simulink model "autopilot_waypoint_mission"  (R2025b)
settings: Solver=FixedStepAuto  StartTime=0.0  StopTime=400  FixedStep=0.01  RelTol=1e-3
InitFcn:
  | %% environmental parameter
  | 
  | g = 9.81;                       %[m/ss]
  | 
  | %% Vehicle parameter
  | 
  | mass = 1.5;                     %[kg]
  | Arm_Length = 0.225;             %[m]
  | 
  | %% Motor parameter
  | 
  | rad2rpm = 60 / (2 * pi);
  | 
  | rpm2rad = 1 / rad2rpm;
  | 
  | Friction_Coef = 0.0001;         %[N m /s]
  | 
  | Inertia = 2.8e-05;              %[kg m^2]
  | 
  | Resistance = 0.1170;            %[ohm]
  | 
  | K_Torque = 1 / (rpm2rad * 960); %[N m/A]
  | 
  | K_Emf = K_Torque;               %[V s/rad]
  | 
  | tau = (Inertia * Resistance) / (Resistance * Friction_Coef + K_Torque * K_Emf);
  | 
  | k_s = K_Torque / (Resistance * Friction_Coef + K_Torque * K_Emf);
  | 
  | Thrust_Coef = 1.1768e-05;
  | 
  | Drag_Coef = 1.8542e-07;
  | 
  | Hovering_Motor_Speed = sqrt(mass * g / (4 * Thrust_Coef));
  | 
  | k_p = 1/k_s;
  | 
  | K1_ALT = 2.1;
  | K2_ALT = 0.7142;
  | 
  | K1_POS = 1.26;
  | K2_POS = 0.4286;
libraries: simulink_extras x8, uavutilslib x1
settings Model: Creator=user  LastModifiedBy=user

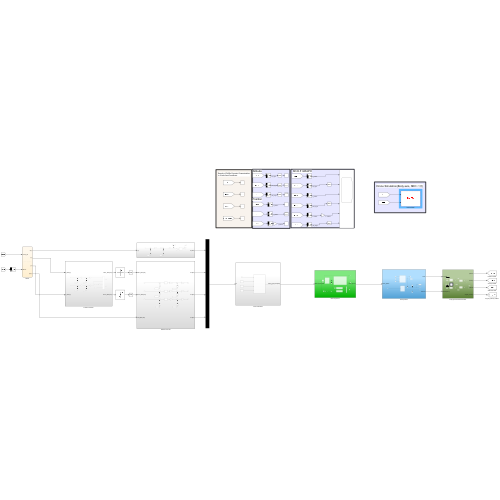
[thumbnail: Simulink's stored preview of the top-level diagram]
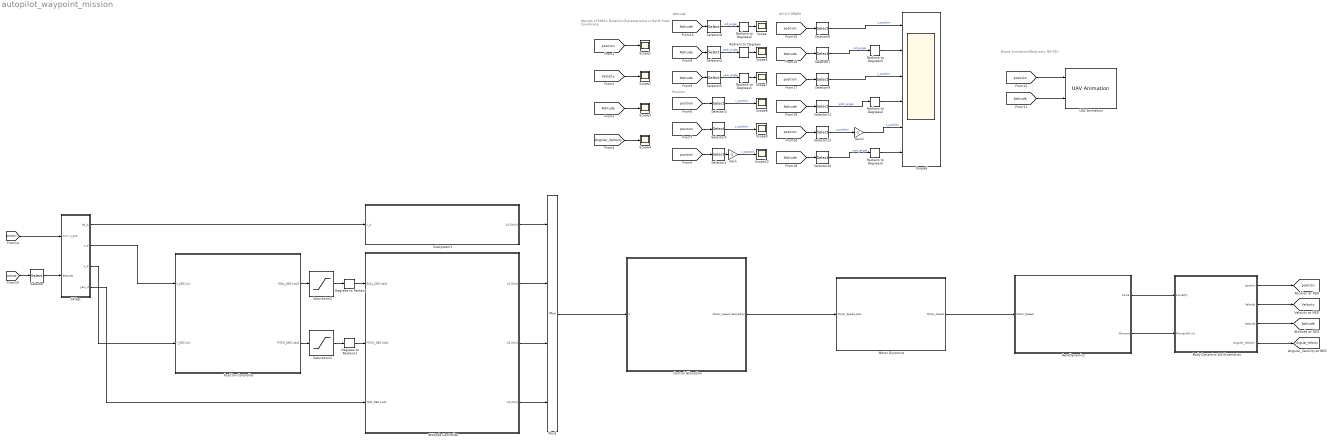
== system autopilot_waypoint_mission ==
  note: Attitude
  note: Results of F450's Dynamic Characteristics
      | in Earth fixed Coordinate
  note: Position
  note: 6D.O.F GRAPH
  note: Drone Simulation(Body axis, NED 기준)
  AeroDynamics : Subsystem
  Attitude Controller : Subsystem
  Body Dynamics && Kinematics : Subsystem
  Control Allocation : Subsystem
  Degrees to Radians : simulink_extras/Transformations/Degrees to Radians
  Degrees to Radians1 : simulink_extras/Transformations/Degrees to Radians
  Gain : Gain  Gain=-1
  Gain1 : Gain  Gain=-1
  Motor Dynamics : Subsystem
  Mux1 : Mux
  Position Controller : Subsystem
  Radians to Degrees{,1..5} (6 alike) : simulink_extras/Transformations/Radians to Degrees
  SP Set : Stateflow chart  TreatAsAtomicUnit=on
      settings: PortSchema="{\"entries\":[{\"content\":{\"sides\":[{\"content\":{},\"type\":\"ConnectorPlacement.EquallySpacedRectSide\",\"uuid\":\"3e53484f-0db2-495f-837b-267abd105f28\"},{\"content\":{\"side\":\"RIGHT\"},\"type\":\"ConnectorPlacement.EquallySpacedRectSide\",\"uuid\":\"c216aad6-ad66-4255-85c0-6c38f2606c75\"},{\"content\":{\"connectorIds\":[\"In2\",\"In1\"],\"side\":\"TOP\"},\"type\":\"ConnectorPlacement.EquallySpacedRectSide\",\"uuid\":\"2b1aea76-ce92-43d3-9c38-2c398ee5c197\"},{\"content\":{\"connectorIds\":[\"Out4\",\"Out2\",\"Out1\",\"Out3\"],\"side\":\"BOTTOM\"},\"type\":\"ConnectorPlacement.EquallySpacedRectSide\",\"uuid\":\"b9774cfe-4d99-465a-9e54-dae465952399\"}]},\"type\":\"ConnectorPlacement.EquallySpacedConnector\",\"uuid\":\"ddf8ca19-aa2c-423c-a9ec-aafb509ad8aa\"}],\"packageUris\":[\"http://schema.mathworks.com/mf0/Connector/R2020b\"],\"version\":\"1.0\"}"
  Saturation1 : Saturate  UpperLimit=30  LowerLimit=-30
  Saturation2 : Saturate  UpperLimit=30  LowerLimit=-30
  Scope{,1..5,7..10} (10 alike) : Scope
      Scope1 settings: Title=Position  ActiveDisplayYMinimum=-2599.70657  ActiveDisplayYMaximum=308.02028  YLabel=[m]  DataLoggingVariableName=ScopeData2
      Scope10 settings: DataLoggingVariableName=ScopeData6
      Scope2 settings: Title=Velocity  ActiveDisplayYMinimum=-56.12917  ActiveDisplayYMaximum=85.41613  YLabel=[m/s]  DataLoggingVariableName=ScopeData3
      Scope3 settings: Title=Attitude  ActiveDisplayYMinimum=-0.68224  ActiveDisplayYMaximum=0.69065  YLabel=[rad]
      Scope4 settings: Title=Angular_Velocity  ActiveDisplayYMinimum=-2.51743  ActiveDisplayYMaximum=2.43948  YLabel=[rad/s]  DataLoggingVariableName=ScopeData2
      Scope5 settings: DataLoggingVariableName=ScopeData2
      Scope7 settings: ActiveDisplayYMinimum=-114.67339  ActiveDisplayYMaximum=12.74149  DataLoggingVariableName=ScopeData3
      Scope8 settings: DataLoggingVariableName=ScopeData4
      Scope9 settings: DataLoggingVariableName=ScopeData5
  Scope6 : Scope  NumInputPorts=6
      settings: ActiveDisplayYMinimum=-3713.64731  ActiveDisplayYMaximum=1009.89473
  Selector : Selector  InputPortWidth=3  IndexOptions=Index vector (dialog)  Indices=3  OutputSizes=1
  Selector{1,5,9..10} (4 alike) : Selector  InputPortWidth=3  IndexOptions=Index vector (dialog)  Indices=[3]  OutputSizes=1
  Selector{2,6,8,11} (4 alike) : Selector  InputPortWidth=3  IndexOptions=Index vector (dialog)  Indices=1  OutputSizes=1
  Selector12 : Selector  InputPortWidth=3  IndexOptions=Index vector (dialog)  Indices=3  OutputSizes=1
  Selector3 : Selector  InputPortWidth=3  IndexOptions=Index vector (dialog)  Indices=2  OutputSizes=1
  Selector4 : Selector  InputPortWidth=3  IndexOptions=Index vector (dialog)  Indices=2  OutputSizes=1
  Selector7 : Selector  InputPortWidth=3  IndexOptions=Index vector (dialog)  Indices=2  OutputSizes=1
  Subsystem1 : Subsystem
  UAV Animation : uavutilslib/UAV Animation  NumUAV=1  DynamicUAVConfig=off  UAVType=Multirotor  UAVSize=1  UAVColor=[1 0 0]  UAVTrajectoryAlpha=1  InertialZDirection=Down  RotationFormat=Euler ZYX  DrawMarkers=off  SampleTime=0.1
  tag scope: Angular_Velocity=global, Attitude=global, Velocity=global, position=global
  wires:
  Motor Dynamics/1(Motor_Speed) -> AeroDynamics/1(Motor_Speed)
  Body Dynamics && Kinematics/3(attitude) -> [Attitude]
  Body Dynamics && Kinematics/1(position) -> [position]
  [Velocity] -> Scope2/1
  [position] -> Scope1/1
  AeroDynamics/1(Force) -> Body Dynamics && Kinematics/1(Force[N])
  AeroDynamics/2(Moment) -> Body Dynamics && Kinematics/2(Moment[N m])
  Body Dynamics && Kinematics/2(Velocity) -> [Velocity]
  Body Dynamics && Kinematics/4(Angular_Velocity) -> [Angular_Velocity]
  [Attitude] -> Scope3/1
  [Angular_Velocity] -> Scope4/1
  Control Allocation/1(Motor_speed_des[rad/s]) -> Motor Dynamics/1(Motor_Speed_Des)
  Mux1/1 -> Control Allocation/1(U)
  [Attitude] -> Selector8/1
  Attitude Controller/1(U2 [Nm]) -> Mux1/2
  Attitude Controller/2(U3 [Nm]) -> Mux1/3
  Attitude Controller/3(U4 [Nm]) -> Mux1/4
  Subsystem1/1(U1 [N/m]) -> Mux1/1
  Selector1/1 -> Gain/1
  [position] -> Selector1/1
  Position Controller/1(ROLL_DES [rad]) -> Saturation2/1
  Position Controller/2(PITCH_DES [rad]) -> Saturation1/1
  [position] -> Selector2/1
  [position] -> Selector3/1
  [Attitude] -> Selector4/1
  [Attitude] -> Selector5/1
  Saturation1/1 -> Degrees to Radians1/1
  Degrees to Radians1/1 -> Attitude Controller/2(PITCH_DES [rad])
  Saturation2/1 -> Degrees to Radians/1
  Degrees to Radians/1 -> Attitude Controller/1(ROLL_DES [rad])
  SP Set/3(alt_d) -> Subsystem1/1(x_d)
  SP Set/1(x_d) -> Position Controller/1(X_DES [m])
  SP Set/2(y_d) -> Position Controller/2(Y_DES [m])
  SP Set/4(yaw_d) -> Attitude Controller/3(YAW_DES [rad])
  [position] -> SP Set/1(current_pos)
  [Attitude] -> Selector/1
  Selector/1 -> SP Set/2(attitude)
  [position] -> UAV Animation/1
  [Attitude] -> UAV Animation/2
  Selector8/1 -> Radians to Degrees2/1  "roll_angle"
  Selector4/1 -> Radians to Degrees/1  "pitch_angle"
  Selector5/1 -> Radians to Degrees1/1  "yaw_angle"
  Selector2/1 -> Scope8/1  "x_position"
  Selector3/1 -> Scope9/1  "y_position"
  Gain/1 -> Scope10/1  "z_position"
  Selector6/1 -> Scope6/1  "x_position"
  [position] -> Selector6/1
  Selector9/1 -> Scope6/3  "y_position"
  Selector7/1 -> Radians to Degrees3/1  "roll_angle"
  [position] -> Selector9/1
  [Attitude] -> Selector7/1
  Selector12/1 -> Gain1/1  "z_position"
  Selector10/1 -> Radians to Degrees5/1  "yaw_angle"
  Selector11/1 -> Radians to Degrees4/1  "pitch_angle"
  [Attitude] -> Selector10/1
  [position] -> Selector12/1
  [Attitude] -> Selector11/1
  Gain1/1 -> Scope6/5  "z_position"
  Radians to Degrees/1 -> Scope5/1
  Radians to Degrees1/1 -> Scope7/1
  Radians to Degrees2/1 -> Scope/1
  Radians to Degrees3/1 -> Scope6/2
  Radians to Degrees4/1 -> Scope6/4
  Radians to Degrees5/1 -> Scope6/6

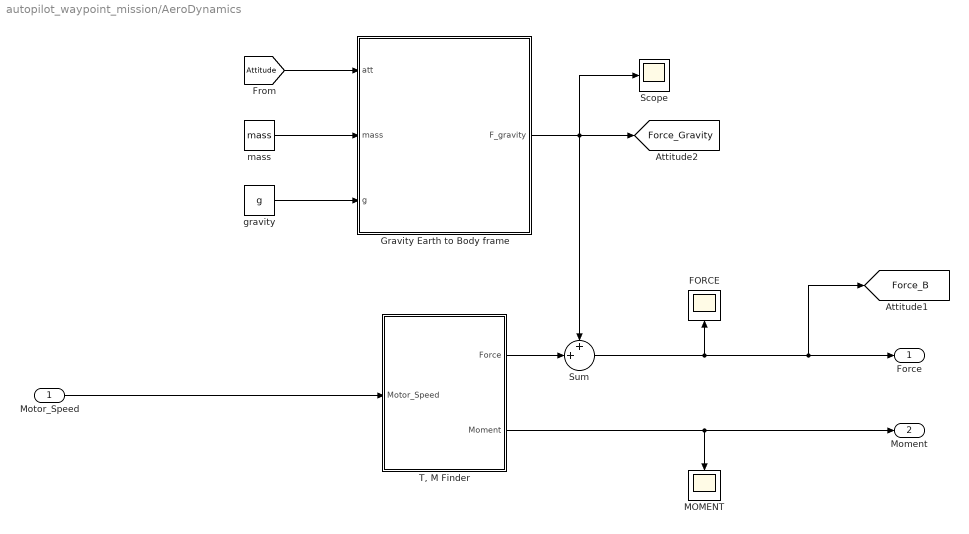
== system autopilot_waypoint_mission/AeroDynamics ==
  Motor_Speed : Inport
  FORCE : Scope
      settings: Title=Body Force Net  ActiveDisplayYMinimum=-2.48819  ActiveDisplayYMaximum=16.62647  YLabel=Force [N]  DataLoggingVariableName=ScopeData4
  Gravity Earth to Body frame : MATLAB Function  TreatAsAtomicUnit=on
  MOMENT : Scope
      settings: ActiveDisplayYMinimum=-0.01497  ActiveDisplayYMaximum=0.13326  DataLoggingVariableName=ScopeData5
  Scope : Scope
      settings: Title=Force_gravity in NED  ActiveDisplayYMinimum=-1.83938  ActiveDisplayYMaximum=16.55438  YLabel=Force [N]
  Sum : Sum  Inputs=++|
  "T, M Finder" : MATLAB Function  TreatAsAtomicUnit=on
  gravity : Constant  Value=g
  mass : Constant  Value=mass
  Force : Outport
  Moment : Outport  Port=2
  tag scope: Force_B=global, Force_Gravity=global
  wires:
  [Attitude] -> Gravity Earth to Body frame/1(att)
  Gravity Earth to Body frame/1(F_gravity) -> Scope/1, [Force_Gravity], Sum/1
  Motor_Speed/1 -> "T, M Finder"/1(Motor_Speed)
  mass/1 -> Gravity Earth to Body frame/2(mass)
  "T, M Finder"/1(Force) -> Sum/2
  gravity/1 -> Gravity Earth to Body frame/3(g)
  Sum/1 -> [Force_B], Force/1, FORCE/1
  "T, M Finder"/2(Moment) -> Moment/1, MOMENT/1

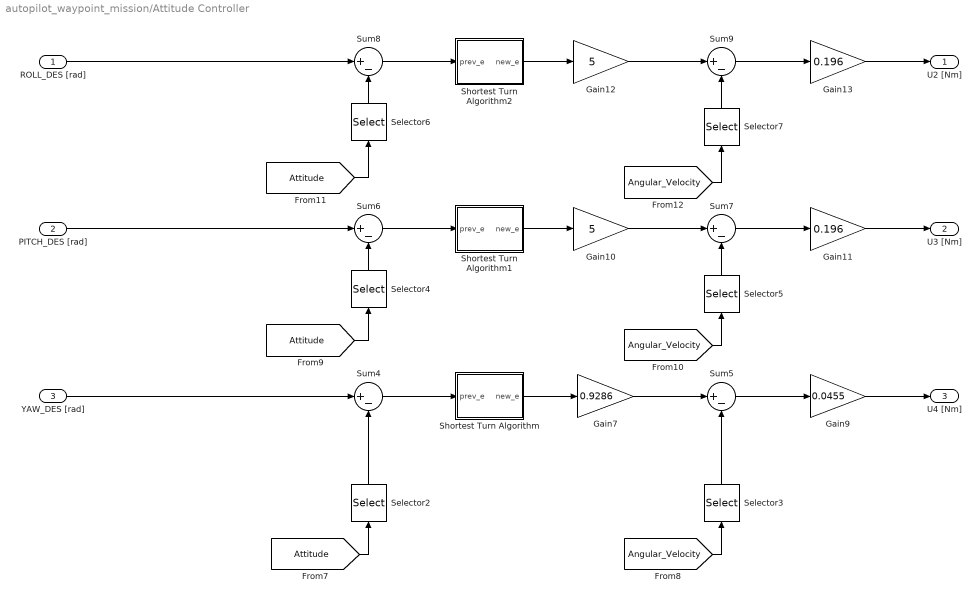
== system autopilot_waypoint_mission/Attitude Controller ==
  ROLL_DES [rad] : Inport
  PITCH_DES [rad] : Inport  Port=2
  YAW_DES [rad] : Inport  Port=3
  Gain10 : Gain  Gain=5
  Gain11 : Gain  Gain=0.196
  Gain12 : Gain  Gain=5
  Gain13 : Gain  Gain=0.196
  Gain7 : Gain  Gain=0.9286
  Gain9 : Gain  Gain=0.0455
  Selector2 : Selector  InputPortWidth=3  IndexOptions=Index vector (dialog)  Indices=[3]  OutputSizes=1
  Selector3 : Selector  InputPortWidth=3  IndexOptions=Index vector (dialog)  Indices=[3]  OutputSizes=1
  Selector4 : Selector  InputPortWidth=3  IndexOptions=Index vector (dialog)  Indices=[2]  OutputSizes=1
  Selector5 : Selector  InputPortWidth=3  IndexOptions=Index vector (dialog)  Indices=[2]  OutputSizes=1
  Selector6 : Selector  InputPortWidth=3  IndexOptions=Index vector (dialog)  Indices=[1]  OutputSizes=1
  Selector7 : Selector  InputPortWidth=3  IndexOptions=Index vector (dialog)  Indices=[1]  OutputSizes=1
  Shortest Turn Algorithm : MATLAB Function  TreatAsAtomicUnit=on
  Shortest Turn Algorithm1 : MATLAB Function  TreatAsAtomicUnit=on
  Shortest Turn Algorithm2 : MATLAB Function  TreatAsAtomicUnit=on
  Sum{4..9} (6 alike) : Sum  Inputs=|+-
  U2 [Nm] : Outport
  U3 [Nm] : Outport  Port=2
  U4 [Nm] : Outport  Port=3
  wires:
  Shortest Turn Algorithm/1(new_e) -> Gain7/1
  Gain9/1 -> U4 [Nm]/1
  [Attitude] -> Selector4/1
  Selector4/1 -> Sum6/2
  [Angular_Velocity] -> Selector3/1
  Gain7/1 -> Sum5/1
  Selector6/1 -> Sum8/2
  Sum9/1 -> Gain13/1
  Gain12/1 -> Sum9/1
  Gain10/1 -> Sum7/1
  Selector5/1 -> Sum7/2
  Sum4/1 -> Shortest Turn Algorithm/1(prev_e)
  [Angular_Velocity] -> Selector7/1
  Sum7/1 -> Gain11/1
  PITCH_DES [rad]/1 -> Sum6/1
  Selector2/1 -> Sum4/2
  [Angular_Velocity] -> Selector5/1
  Gain11/1 -> U3 [Nm]/1
  Selector3/1 -> Sum5/2
  [Attitude] -> Selector6/1
  ROLL_DES [rad]/1 -> Sum8/1
  [Attitude] -> Selector2/1
  Sum5/1 -> Gain9/1
  Selector7/1 -> Sum9/2
  YAW_DES [rad]/1 -> Sum4/1
  Gain13/1 -> U2 [Nm]/1
  Sum8/1 -> Shortest Turn Algorithm2/1(prev_e)
  Shortest Turn Algorithm2/1(new_e) -> Gain12/1
  Sum6/1 -> Shortest Turn Algorithm1/1(prev_e)
  Shortest Turn Algorithm1/1(new_e) -> Gain10/1

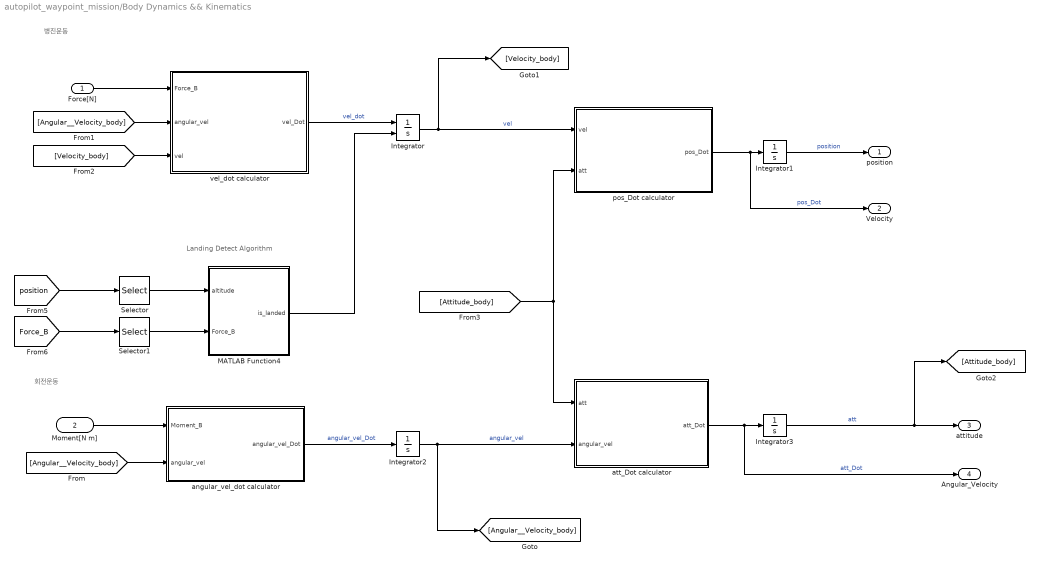
== system autopilot_waypoint_mission/Body Dynamics && Kinematics ==
  note: 병진운동
  note: 회전운동
  note: Landing Detect Algorithm
  Force[N] : Inport
  Moment[N m] : Inport  Port=2
  Integrator : Integrator  ExternalReset=level hold  InitialCondition=[0 0 0]'
  Integrator1 : Integrator  InitialCondition=[0 0 0]'  LimitOutput=on  UpperSaturationLimit=[inf inf 0]'  LowerSaturationLimit=[-inf -inf -inf]'  ZeroCross=off
  Integrator2 : Integrator  InitialCondition=[0 0 0]'
  Integrator3 : Integrator  InitialCondition=[0 0 0]'  WrapState=on
  MATLAB Function4 : MATLAB Function  TreatAsAtomicUnit=on
  Selector : Selector  InputPortWidth=3  IndexOptions=Index vector (dialog)  Indices=[3]  OutputSizes=1
  Selector1 : Selector  InputPortWidth=3  IndexOptions=Index vector (dialog)  Indices=[3]  OutputSizes=1
  angular_vel_dot calculator : MATLAB Function  TreatAsAtomicUnit=on
  att_Dot calculator : MATLAB Function  TreatAsAtomicUnit=on
  pos_Dot calculator : MATLAB Function  TreatAsAtomicUnit=on
  vel_dot calculator : MATLAB Function  TreatAsAtomicUnit=on
  position : Outport
  Velocity : Outport  Port=2
  attitude : Outport  Port=3
  Angular_Velocity : Outport  Port=4
  wires:
  Force[N]/1 -> vel_dot calculator/1(Force_B)
  Moment[N m]/1 -> angular_vel_dot calculator/1(Moment_B)
  Integrator/1 -> pos_Dot calculator/1(vel), [Velocity_body]  "vel"
  pos_Dot calculator/1(pos_Dot) -> Velocity/1, Integrator1/1  "pos_Dot"
  Integrator1/1 -> position/1  "position"
  Integrator2/1 -> att_Dot calculator/2(angular_vel), [Angular__Velocity_body]  "angular_vel"
  Integrator3/1 -> attitude/1, [Attitude_body]  "att"
  att_Dot calculator/1(att_Dot) -> Angular_Velocity/1, Integrator3/1  "att_Dot"
  [Angular__Velocity_body] -> angular_vel_dot calculator/2(angular_vel)
  [Angular__Velocity_body] -> vel_dot calculator/2(angular_vel)
  [Velocity_body] -> vel_dot calculator/3(vel)
  [Attitude_body] -> pos_Dot calculator/2(att), att_Dot calculator/1(att)
  angular_vel_dot calculator/1(angular_vel_Dot) -> Integrator2/1  "angular_vel_Dot"
  vel_dot calculator/1(vel_Dot) -> Integrator/1  "vel_dot"
  MATLAB Function4/1(is_landed) -> Integrator/2
  Selector1/1 -> MATLAB Function4/2(Force_B)
  [position] -> Selector/1
  [Force_B] -> Selector1/1
  Selector/1 -> MATLAB Function4/1(altitude)

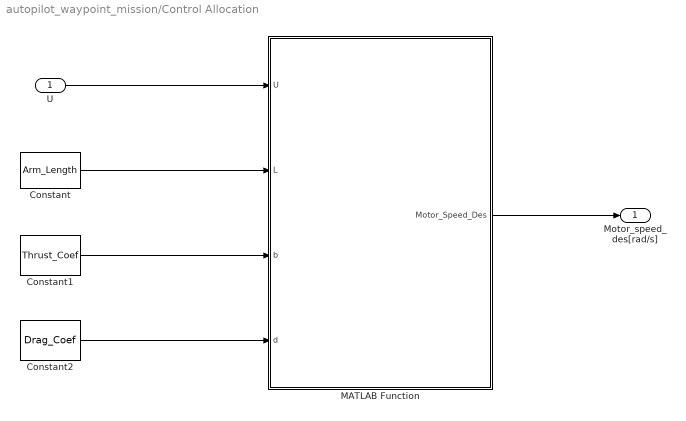
== system autopilot_waypoint_mission/Control Allocation ==
  U : Inport
  Constant : Constant  Value=Arm_Length
  Constant1 : Constant  Value=Thrust_Coef
  Constant2 : Constant  Value=Drag_Coef
  MATLAB Function : MATLAB Function  TreatAsAtomicUnit=on
  Motor_speed_des[rad/s] : Outport
  wires:
  Constant2/1 -> MATLAB Function/4(d)
  MATLAB Function/1(Motor_Speed_Des) -> Motor_speed_des[rad/s]/1
  Constant1/1 -> MATLAB Function/3(b)
  Constant/1 -> MATLAB Function/2(L)
  U/1 -> MATLAB Function/1(U)

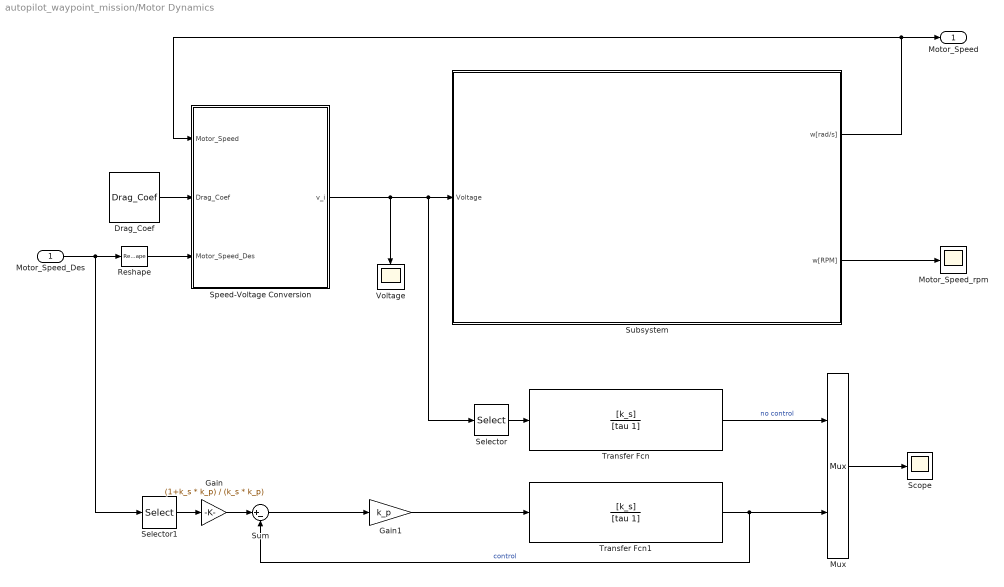
== system autopilot_waypoint_mission/Motor Dynamics ==
  Motor_Speed_Des : Inport
  Drag_Coef : Constant  Value=Drag_Coef
  Gain : Gain  Gain=(1+k_s * k_p) / (k_s * k_p)
  Gain1 : Gain  Gain=k_p
  Motor_Speed_rpm : Scope
      settings: Title=Motor_Speed[Lec2]  ActiveDisplayYMinimum=-1287.7868  ActiveDisplayYMaximum=5339.1248  YLabel=[RPM]
  Mux : Mux  Inputs=2
  Reshape : Reshape  OutputDimensionality=Column vector (2-D)
  Scope : Scope
      settings: ActiveDisplayYMinimum=-69.59196  ActiveDisplayYMaximum=626.32767
  Selector : Selector  InputPortWidth=4  IndexOptions=Index vector (dialog)  Indices=1  OutputSizes=1
  Selector1 : Selector  InputPortWidth=4  IndexOptions=Index vector (dialog)  Indices=1  OutputSizes=1
  Speed-Voltage Conversion : MATLAB Function  TreatAsAtomicUnit=on
  Subsystem : Subsystem
  Sum : Sum  Inputs=|+-
  Transfer Fcn : TransferFcn  Numerator=[k_s]  Denominator=[tau 1]
  Transfer Fcn1 : TransferFcn  Numerator=[k_s]  Denominator=[tau 1]
  Voltage : Scope
      settings: Title=Voltage[Lec2]  ActiveDisplayYMinimum=5.3597  ActiveDisplayYMaximum=7.0724  YLabel=[V]  DataLoggingVariableName=ScopeData2
  Motor_Speed : Outport
  wires:
  Speed-Voltage Conversion/1(v_i) -> Voltage/1, Subsystem/1(Voltage), Selector/1
  Drag_Coef/1 -> Speed-Voltage Conversion/2(Drag_Coef)
  Subsystem/1(w[rad/s]) -> Motor_Speed/1, Speed-Voltage Conversion/1(Motor_Speed)
  Subsystem/2(w[RPM]) -> Motor_Speed_rpm/1
  Motor_Speed_Des/1 -> Selector1/1, Reshape/1
  Reshape/1 -> Speed-Voltage Conversion/3(Motor_Speed_Des)
  Selector/1 -> Transfer Fcn/1
  Selector1/1 -> Gain/1
  Sum/1 -> Gain1/1
  Transfer Fcn1/1 -> Sum/2, Mux/2  "control"
  Gain/1 -> Sum/1
  Gain1/1 -> Transfer Fcn1/1
  Mux/1 -> Scope/1
  Transfer Fcn/1 -> Mux/1  "no control"

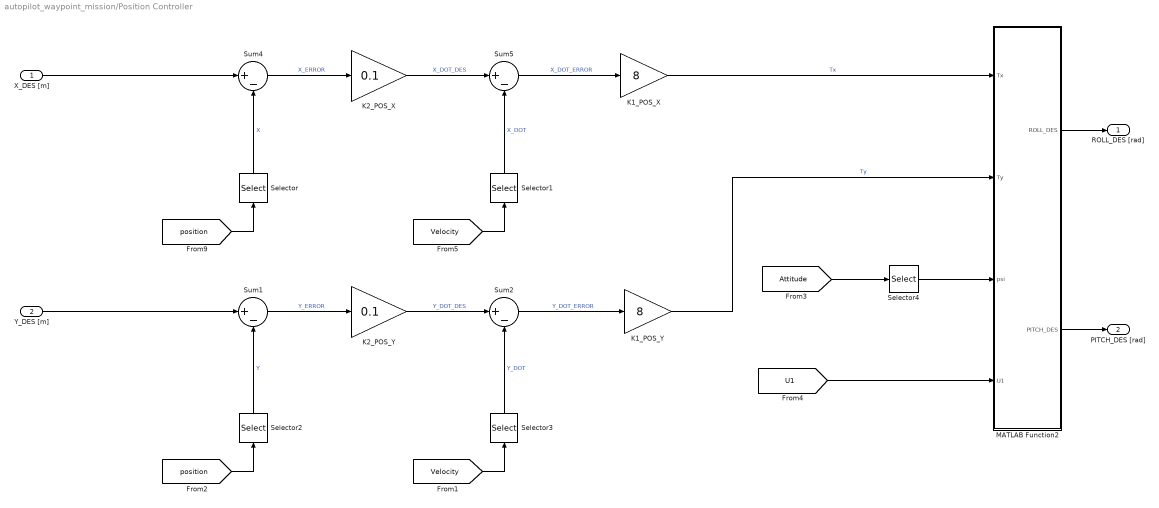
== system autopilot_waypoint_mission/Position Controller ==
  X_DES [m] : Inport
  Y_DES [m] : Inport  Port=2
  K1_POS_X : Gain  Gain=8
  K1_POS_Y : Gain  Gain=8
  K2_POS_X : Gain  Gain=0.1
  K2_POS_Y : Gain  Gain=0.1
  MATLAB Function2 : MATLAB Function  TreatAsAtomicUnit=on
  Selector : Selector  InputPortWidth=3  IndexOptions=Index vector (dialog)  Indices=1  OutputSizes=1
  Selector1 : Selector  InputPortWidth=3  IndexOptions=Index vector (dialog)  Indices=1  OutputSizes=1
  Selector2 : Selector  InputPortWidth=3  IndexOptions=Index vector (dialog)  Indices=2  OutputSizes=1
  Selector3 : Selector  InputPortWidth=3  IndexOptions=Index vector (dialog)  Indices=2  OutputSizes=1
  Selector4 : Selector  InputPortWidth=3  IndexOptions=Index vector (dialog)  Indices=3  OutputSizes=1
  Sum{1..2,4..5} (4 alike) : Sum  Inputs=|+-
  ROLL_DES [rad] : Outport
  PITCH_DES [rad] : Outport  Port=2
  wires:
  [position] -> Selector/1
  K1_POS_X/1 -> MATLAB Function2/1(Tx)  "Tx"
  X_DES [m]/1 -> Sum4/1
  Selector/1 -> Sum4/2  "X"
  [Velocity] -> Selector1/1
  Sum5/1 -> K1_POS_X/1  "X_DOT_ERROR"
  Selector1/1 -> Sum5/2  "X_DOT"
  K2_POS_X/1 -> Sum5/1  "X_DOT_DES"
  Sum4/1 -> K2_POS_X/1  "X_ERROR"
  [position] -> Selector2/1
  K1_POS_Y/1 -> MATLAB Function2/2(Ty)  "Ty"
  Y_DES [m]/1 -> Sum1/1
  Selector2/1 -> Sum1/2  "Y"
  [Velocity] -> Selector3/1
  Sum2/1 -> K1_POS_Y/1  "Y_DOT_ERROR"
  Selector3/1 -> Sum2/2  "Y_DOT"
  K2_POS_Y/1 -> Sum2/1  "Y_DOT_DES"
  Sum1/1 -> K2_POS_Y/1  "Y_ERROR"
  [Attitude] -> Selector4/1
  Selector4/1 -> MATLAB Function2/3(psi)
  [U1] -> MATLAB Function2/4(U1)
  MATLAB Function2/1(ROLL_DES) -> ROLL_DES [rad]/1
  MATLAB Function2/2(PITCH_DES) -> PITCH_DES [rad]/1

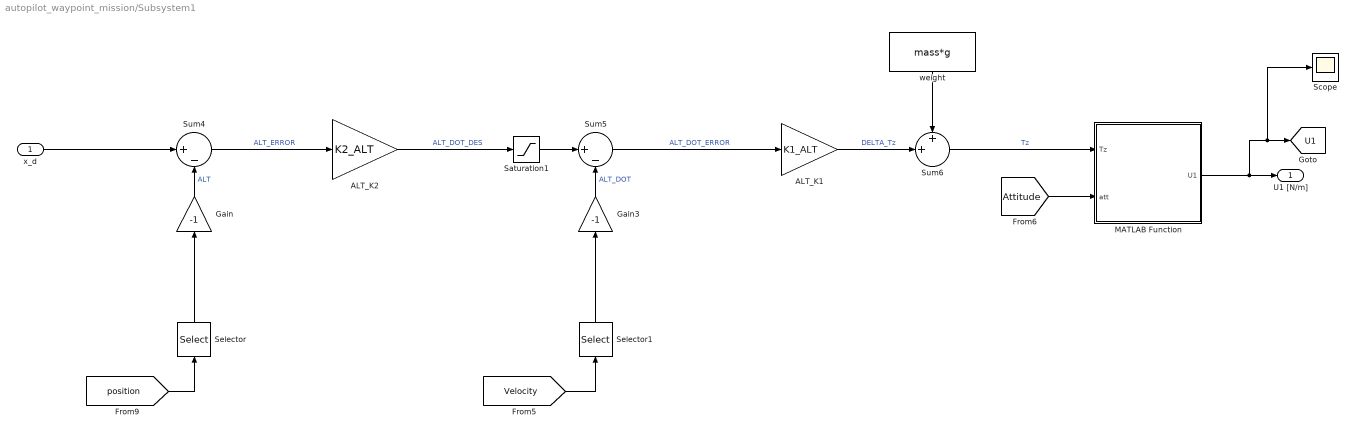
== system autopilot_waypoint_mission/Subsystem1 ==
  x_d : Inport
  ALT_K1 : Gain  Gain=K1_ALT
  ALT_K2 : Gain  Gain=K2_ALT
  Gain : Gain  Gain=-1
  Gain3 : Gain  Gain=-1
  MATLAB Function : MATLAB Function  TreatAsAtomicUnit=on
  Saturation1 : Saturate  UpperLimit=3  LowerLimit=-1.5
  Scope : Scope
      settings: DataLoggingVariableName=ScopeData6
  Selector : Selector  InputPortWidth=3  IndexOptions=Index vector (dialog)  Indices=3  OutputSizes=1
  Selector1 : Selector  InputPortWidth=3  IndexOptions=Index vector (dialog)  Indices=3  OutputSizes=1
  Sum4 : Sum  Inputs=|+-
  Sum5 : Sum  Inputs=|+-
  Sum6 : Sum  Inputs=++|
  weight : Constant  Value=mass*g
  U1 [N/m] : Outport
  tag scope: U1=global
  wires:
  Gain3/1 -> Sum5/2  "ALT_DOT"
  Sum5/1 -> ALT_K1/1  "ALT_DOT_ERROR"
  ALT_K2/1 -> Saturation1/1  "ALT_DOT_DES"
  Sum4/1 -> ALT_K2/1  "ALT_ERROR"
  Sum6/1 -> MATLAB Function/1(Tz)  "Tz"
  weight/1 -> Sum6/1
  ALT_K1/1 -> Sum6/2  "DELTA_Tz"
  Selector1/1 -> Gain3/1
  [position] -> Selector/1
  Gain/1 -> Sum4/2  "ALT"
  Selector/1 -> Gain/1
  [Velocity] -> Selector1/1
  [Attitude] -> MATLAB Function/2(att)
  MATLAB Function/1(U1) -> Scope/1, [U1], U1 [N/m]/1
  x_d/1 -> Sum4/1
  Saturation1/1 -> Sum5/1

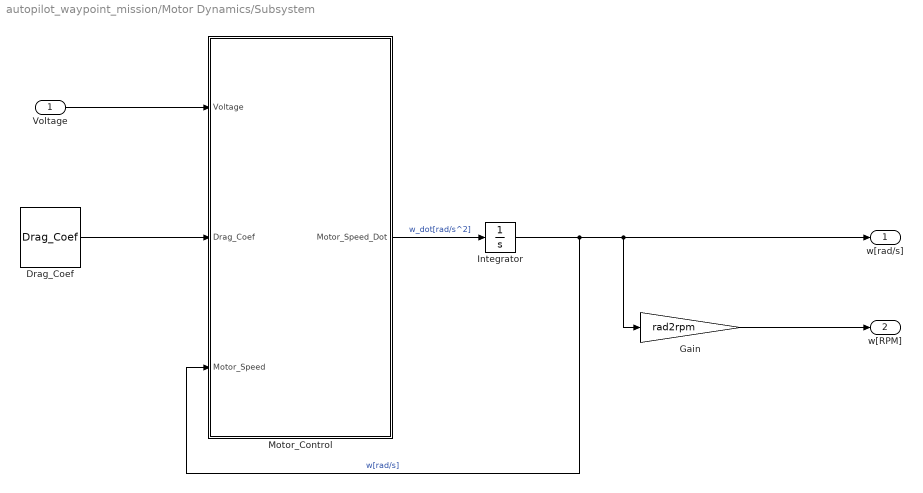
== system autopilot_waypoint_mission/Motor Dynamics/Subsystem ==
  Voltage : Inport
  Drag_Coef : Constant  Value=Drag_Coef
  Gain : Gain  Gain=rad2rpm
  Integrator : Integrator  InitialCondition=[0 0 0 0]'
  Motor_Control : MATLAB Function  TreatAsAtomicUnit=on
  w[rad/s] : Outport
  w[RPM] : Outport  Port=2
  wires:
  Motor_Control/1(Motor_Speed_Dot) -> Integrator/1  "w_dot[rad/s^2]"
  Integrator/1 -> w[rad/s]/1, Gain/1, Motor_Control/3(Motor_Speed)  "w[rad/s]"
  Gain/1 -> w[RPM]/1
  Voltage/1 -> Motor_Control/1(Voltage)
  Drag_Coef/1 -> Motor_Control/2(Drag_Coef)

== matlab function autopilot_waypoint_mission/Body Dynamics && Kinematics/vel_dot calculator ==
  data: Force_B input; vel_Dot output; angular_vel input; vel input
function vel_Dot = fcn(Force_B, angular_vel, vel)
mass = 1.5;
vel_Dot = Force_B / mass - cross(angular_vel, vel);

== matlab function autopilot_waypoint_mission/Body Dynamics && Kinematics/angular_vel_dot calculator ==
  data: Moment_B input; angular_vel_Dot output; angular_vel input
function angular_vel_Dot = fcn(Moment_B, angular_vel)

Inertia = diag([0.02 0.02 0.025]);

angular_vel_Dot = Inertia ^ (-1) * (Moment_B - cross(angular_vel, Inertia * angular_vel));

== matlab function autopilot_waypoint_mission/Body Dynamics && Kinematics/pos_Dot calculator ==
  data: vel input; pos_Dot output; att input
function pos_Dot = fcn(vel, att)
%바디축의 velocity

phi = att(1);
theta = att(2);
psi = att(3);

c_psi = cos(psi);
s_psi = sin(psi);
c_theta = cos(theta);
s_theta = sin(theta);
c_phi = cos(phi);
s_phi = sin(phi);


%R_EB
R_B2E = [c_psi*c_theta      c_psi*s_theta*s_phi-s_psi*c_phi         c_psi*s_theta*c_phi + s_psi*s_phi;
        s_psi*c_theta       s_psi*s_theta*s_phi + c_psi*c_phi       s_psi*s_theta*c_phi - c_psi*s_phi;
           -s_theta                 c_theta*s_phi                               c_theta*c_phi];



pos_Dot = R_B2E * vel;

== matlab function autopilot_waypoint_mission/Body Dynamics && Kinematics/att_Dot calculator ==
  data: att input; angular_vel input; att_Dot output
function att_Dot = fcn(att, angular_vel)

phi = att(1);
theta = att(2);



R_B2E = [1      sin(phi)*tan(theta)     cos(phi)*tan(theta);
         0              cos(phi)            -sin(phi);
         0      sin(phi)*sec(theta)     cos(phi)*sec(theta)];


att_Dot = R_B2E * angular_vel;

== matlab function autopilot_waypoint_mission/Body Dynamics && Kinematics/MATLAB Function4 ==
  data: is_landed output; altitude input; Force_B input
function is_landed = fcn(altitude, Force_B)

is_landed = (altitude >= 0) && (Force_B > 0);

end

== matlab function autopilot_waypoint_mission/Attitude Controller/Shortest Turn Algorithm ==
  data: prev_e input; new_e output
function new_e = fcn(prev_e)

if prev_e > pi
    new_e = prev_e - 2 * pi;
elseif prev_e < -pi
    new_e = prev_e + 2 * pi;
else
    new_e = prev_e;
end

== matlab function autopilot_waypoint_mission/Attitude Controller/Shortest Turn Algorithm1 ==
  data: prev_e input; new_e output
function new_e = fcn(prev_e)

if prev_e > pi
    new_e = prev_e - 2 * pi;
elseif prev_e < -pi
    new_e = prev_e + 2 * pi;
else
    new_e = prev_e;
end

== matlab function autopilot_waypoint_mission/Attitude Controller/Shortest Turn Algorithm2 ==
  data: prev_e input; new_e output
function new_e = fcn(prev_e)

if prev_e > pi
    new_e = prev_e - 2 * pi;
elseif prev_e < -pi
    new_e = prev_e + 2 * pi;
else
    new_e = prev_e;
end

== matlab function autopilot_waypoint_mission/Control Allocation/MATLAB Function ==
  data: U input; Motor_Speed_Des output; L input; b input; d input
function Motor_Speed_Des = fcn(U, L, b, d)

lb = L*b/sqrt(2);


%Arm이 +일 때
%AC = [b  b  b  b;
%      0 -lb 0 lb;
%      lb 0 -lb 0;
%      -d d -d d] ^ (-1);


%Arm이 x일 때
AC = [b  b  b  b;
      -lb lb lb -lb;
      lb -lb lb -lb;
      d d -d -d] ^ (-1);

Motor_Speed_Des_2 = max(AC * U, 0);

Motor_Speed_Des = sqrt(Motor_Speed_Des_2);

== matlab function autopilot_waypoint_mission/Subsystem1/MATLAB Function ==
  data: Tz input; U1 output; att input
function U1 = fcn(Tz, att)

phi = att(1);
theta = att(2);

U1 = Tz / (cos(phi) * cos(theta));

end

== matlab function autopilot_waypoint_mission/Position Controller/MATLAB Function2 ==
  data: Tx input; ROLL_DES output; Ty input; psi input; U1 input; PITCH_DES output
function [ROLL_DES, PITCH_DES] = fcn(Tx, Ty, psi, U1)

Txx = Tx * cos(psi) + Ty * sin(psi);     %Tx'
Tyy = -Tx * sin(psi) + Ty * cos(psi);    %Ty'


ROLL_DES = Tyy/U1;
PITCH_DES = -Txx/U1;

== stateflow chart autopilot_waypoint_mission/SP Set ==
  state SP4
    x_d = -2864.4;  % 예시값 (직접 구한 SP4 x좌표)
    y_d = -294;   % 예시값 (직접 구한 SP4 y좌표)
    alt_d =80;
  state SP5
    x_d = 0;
    y_d = 0;
    alt_d = 50;  % 고도 50m로 하강
  state SP6
    x_d = 0;
    y_d = 0;
    alt_d = 0;  % 고도 50m로 하강
  state Head1
    yaw_d=atan2(-554.4, -73.5);
  state Head2
    yaw_d=atan2(-2864.4 - (-554.4), -294 - (-73.5));
  state Head3
    yaw_d=atan2(0-2864.4, 0 - (-294));
  state SP2
    x_d = 0;
    y_d = 0;
    alt_d = 80;  % 고도 80m
  state SP3
    x_d = -554.4;   % 순리 위도 환산 m
    y_d = -73.5;    % 순리 경도 환산 m
    alt_d = 80;
  note: SP1(Departure)
  SP2 -> Head1 : [[abs(current_pos(3) - (-80)) < 1]]
  Head1 -> SP3 : [abs(yaw_d - attitude) < 0.01]
  SP3 -> Head2 : [norm(current_pos(1:2) - [-554.4; -73.5]) < 1 && abs(current_pos(3) - (-80)) < 1]
  Head2 -> SP4 : [abs(yaw_d - attitude) < 0.01]
  SP4 -> Head3 : [norm(current_pos(1:2) - [-2864.4; -294]) < 1 && abs(current_pos(3) - (-80)) < 1]
  Head3 -> SP5 : [[abs(yaw_d - attitude) < 0.01]]
  SP5 -> SP6 : [abs(current_pos(3) - (-50)) < 1 && norm(current_pos(1:2) - [0; 0]) < 1]
  (default) -> SP2
  data: x_d output; current_pos input; y_d output; alt_d output; yaw_d output; attitude input

== matlab function autopilot_waypoint_mission/Motor Dynamics/Speed-Voltage Conversion ==
  data: Motor_Speed input; Drag_Coef input; Motor_Speed_Des input; v_i output
function v_i = fcn(Motor_Speed, Drag_Coef, Motor_Speed_Des)

rad2rpm = 60 / (2 * pi);

rpm2rad = 1 / rad2rpm;

Resistance = 0.1170;            %[ohm]

K_Torque = 1 / (rpm2rad * 960); %[N m/A]

K_Emf = K_Torque;               %[V s/rad]


v_i = K_Emf .* Motor_Speed_Des + Resistance/K_Torque * Drag_Coef .* Motor_Speed.^2;


end

== matlab function autopilot_waypoint_mission/Motor Dynamics/Subsystem/Motor_Control ==
  data: Voltage input; Drag_Coef input; Motor_Speed_Dot output; Motor_Speed input
function Motor_Speed_Dot = fcn(Voltage, Drag_Coef, Motor_Speed)

rad2rpm = 60 / (2 * pi);

rpm2rad = 1 / rad2rpm;

Inertia = 2.8e-05;              %[kg m^2]

Resistance = 0.1170;            %[ohm]

K_Torque = 1 / (rpm2rad * 960); %[N m/A]

K_Emf = K_Torque;               %[V s/rad]

V_Emf = K_Emf .* Motor_Speed; %[Voltage]

Current = (Voltage - V_Emf) / Resistance; %[A]

Motor_Speed_Dot = (K_Torque * Current - Drag_Coef * Motor_Speed.^2)/ Inertia; %[rad/s^2]

end

== matlab function autopilot_waypoint_mission/AeroDynamics/T, M Finder ==
  data: Motor_Speed input; Force output; Moment output
function [Force, Moment] = fcn(Motor_Speed)

Thrust_Coef = 1.1768e-05;

Drag_Coef = 1.8542e-07;

Arm_Length = 0.225;             %[m]


Force = [0;
         0;
         -Thrust_Coef * sum(Motor_Speed.^2)];


%% Cal Moment
Mx = Arm_Length * Thrust_Coef * (Motor_Speed(3)^2 + Motor_Speed(2)^2 - Motor_Speed(1)^2 -Motor_Speed(4)^2) / sqrt(2);
My = Arm_Length * Thrust_Coef * (Motor_Speed(1)^2 + Motor_Speed(3)^2 - Motor_Speed(2)^2 - Motor_Speed(4)^2) / sqrt(2);
Mz = Drag_Coef * (Motor_Speed(1)^2 + Motor_Speed(2)^2 - Motor_Speed(3)^2 - Motor_Speed(4)^2);

Moment = [Mx; My; Mz];

== matlab function autopilot_waypoint_mission/AeroDynamics/Gravity Earth to Body frame ==
  data: att input; F_gravity output; mass input; g input
function F_gravity = fcn(att, mass, g)

phi = att(1);
theta = att(2);

gravity = g * [-sin(theta);
                sin(phi)*cos(theta);
                cos(phi)*cos(theta)];

F_gravity = mass * gravity;
